simulink model "InductionMachine"  (R2021b)
settings: Solver=FixedStepAuto  StartTime=0.0  StopTime=5  FixedStep=1e-5  RelTol=1e-3
values from neighbouring files (symbols this model uses):
  B = 0.001    [InductionMachine_cal.m]    (also in InductionMachine_dq_cal.m)
  J = 0.2    [InductionMachine_cal.m]    (also in InductionMachine_dq_cal.m)
  L0 = 134.2e-3    (= 0.1342)    [InductionMachine_cal.m]    (also in InductionMachine_dq_cal.m)
  L1 = 135.6e-3    (= 0.1356)    [InductionMachine_cal.m]    (also in InductionMachine_dq_cal.m)
  L2 = 135.6e-3    (= 0.1356)    [InductionMachine_cal.m]    (also in InductionMachine_dq_cal.m)
  omegaSuply = 120 * pi    (= 376.991118431)    [InductionMachine_cal.m]
  P = 4    [InductionMachine_cal.m]    (also in InductionMachine_dq_cal.m)
  R1 = .75    (= 0.75)    [InductionMachine_cal.m]    (also in InductionMachine_dq_cal.m)
  R2 = .46    (= 0.46)    [InductionMachine_cal.m]    (also in InductionMachine_dq_cal.m)
  Tl = 0    [InductionMachine_cal.m]    (also in InductionMachine_dq_cal.m)
  Vsupply = 163    [InductionMachine_cal.m]
Description:
  | Exercise 03 - Lecture 09
settings Model: Creator=Dinh-Tuyen Le  LastModifiedBy=Dinh-Tuyen Le

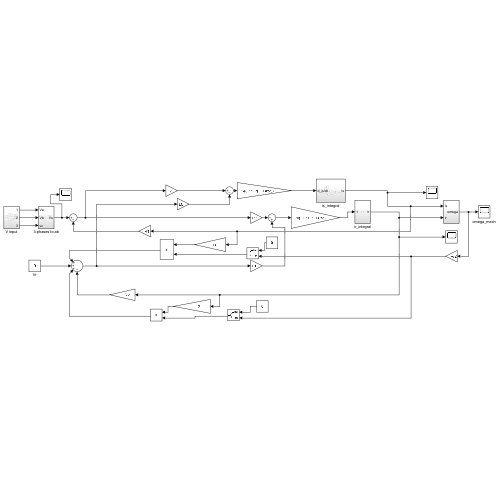
[thumbnail: Simulink's stored preview of the top-level diagram]
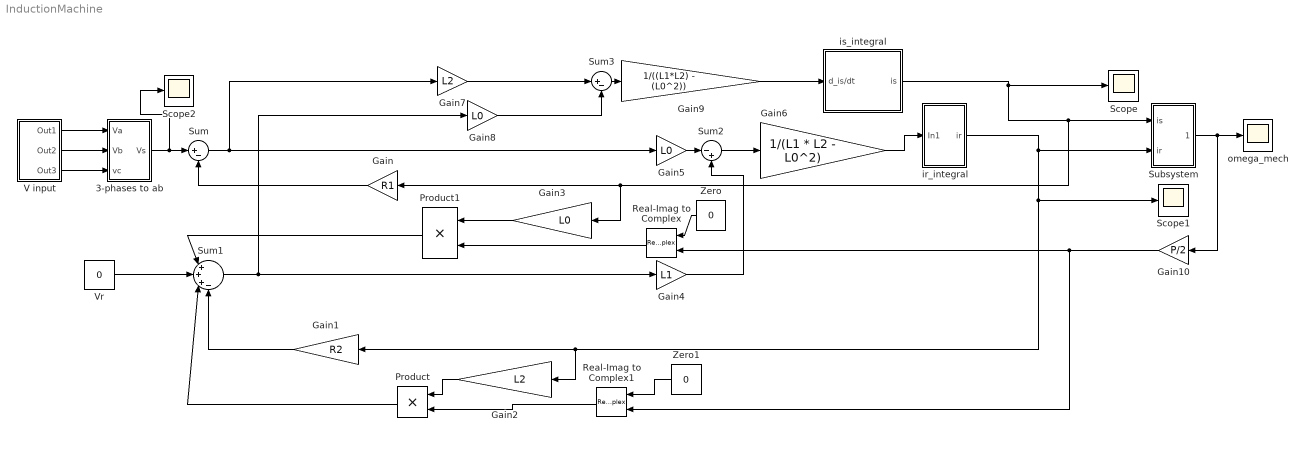
== system InductionMachine ==
  3-phases to ab : Subsystem
  Gain : Gain  Gain=R1
  Gain1 : Gain  Gain=R2
  Gain10 : Gain  Gain=P/2
  Gain2 : Gain  Gain=L2
  Gain3 : Gain  Gain=L0
  Gain4 : Gain  Gain=L1
  Gain5 : Gain  Gain=L0
  Gain6 : Gain  Gain=1/(L1 * L2 - L0^2)
  Gain7 : Gain  Gain=L2
  Gain8 : Gain  Gain=L0
  Gain9 : Gain  Gain=1/((L1*L2) - (L0^2))
  Product : Product
  Product1 : Product
  Real-Imag to Complex : RealImagToComplex
  Real-Imag to Complex1 : RealImagToComplex
  Scope : Scope
  Scope1 : Scope
  Scope2 : Scope
  Subsystem : Subsystem
  Sum : Sum  Inputs=|+-
  Sum1 : Sum  Inputs=|+++-
  Sum2 : Sum  Inputs=|-+
  Sum3 : Sum  Inputs=|+-
  V input : Subsystem
  Vr : Constant  Value=0  OutDataTypeStr=Inherit: Inherit via back propagation
  Zero : Constant  Value=0  OutDataTypeStr=Inherit: Inherit via back propagation
  Zero1 : Constant  Value=0  OutDataTypeStr=Inherit: Inherit via back propagation
  ir_integral : Subsystem
  is_integral : Subsystem
  omega_mech : Scope
  wires:
  Gain/1 -> Sum/2
  Gain1/1 -> Sum1/4
  Vr/1 -> Sum1/2
  Sum1/1 -> Gain8/1, Gain4/1
  Sum/1 -> Gain5/1, Gain7/1
  Gain5/1 -> Sum2/1
  Gain4/1 -> Sum2/2
  Sum2/1 -> Gain6/1
  Gain7/1 -> Sum3/1
  Gain8/1 -> Sum3/2
  Sum3/1 -> Gain9/1
  3-phases to ab/1(Vs) -> Sum/1, Scope2/1
  Subsystem/1(omega) -> omega_mech/1, Gain10/1
  ir_integral/1(ir) -> Gain2/1, Gain1/1, Scope1/1, Subsystem/2(ir)
  Gain6/1 -> ir_integral/1(In1)
  is_integral/1(is) -> Gain/1, Gain3/1, Subsystem/1(is), Scope/1
  Gain9/1 -> is_integral/1(d_is/dt)
  Gain2/1 -> Product/1
  Product/1 -> Sum1/3
  Gain3/1 -> Product1/1
  Product1/1 -> Sum1/1
  Real-Imag to Complex/1 -> Product1/2
  Zero/1 -> Real-Imag to Complex/1
  Zero1/1 -> Real-Imag to Complex1/1
  Real-Imag to Complex1/1 -> Product/2
  V input/1(Out1) -> 3-phases to ab/1(Va)
  V input/2(Out2) -> 3-phases to ab/2(Vb)
  V input/3(Out3) -> 3-phases to ab/3(vc)
  Gain10/1 -> Real-Imag to Complex1/2, Real-Imag to Complex/2

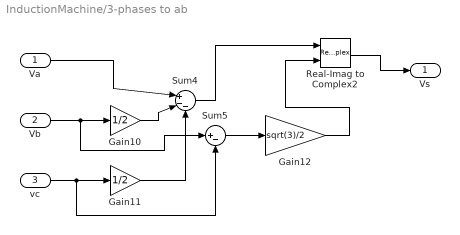
== system InductionMachine/3-phases to ab ==
  Va : Inport
  Vb : Inport  Port=2
  vc : Inport  Port=3
  Gain10 : Gain  Gain=1/2
  Gain11 : Gain  Gain=1/2
  Gain12 : Gain  Gain=sqrt(3)/2
  Real-Imag to Complex2 : RealImagToComplex
  Sum4 : Sum  Inputs=|+--
  Sum5 : Sum  Inputs=|+-
  Vs : Outport
  wires:
  Gain12/1 -> Real-Imag to Complex2/2
  Vb/1 -> Sum5/1, Gain10/1
  Va/1 -> Sum4/1
  Sum4/1 -> Real-Imag to Complex2/1
  Sum5/1 -> Gain12/1
  vc/1 -> Sum5/2, Gain11/1
  Gain11/1 -> Sum4/3
  Gain10/1 -> Sum4/2
  Real-Imag to Complex2/1 -> Vs/1

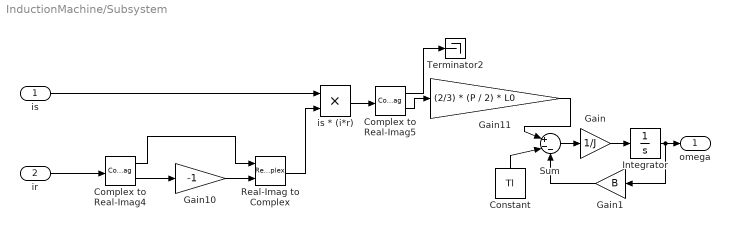
== system InductionMachine/Subsystem ==
  is : Inport
  ir : Inport  Port=2
  Complex to Real-Imag4 : ComplexToRealImag
  Complex to Real-Imag5 : ComplexToRealImag
  Constant : Constant  Value=Tl
  Gain : Gain  Gain=1/J
  Gain1 : Gain  Gain=B
  Gain10 : Gain  Gain=-1
  Gain11 : Gain  Gain=(2/3) * (P / 2) * L0
  Integrator : Integrator
  Real-Imag to Complex : RealImagToComplex
  Sum : Sum  Inputs=|+--
  Terminator2 : Terminator
  is * (i*r) : Product
  omega : Outport
  wires:
  Complex to Real-Imag5/1 -> Terminator2/1
  Complex to Real-Imag5/2 -> Gain11/1
  is * (i*r)/1 -> Complex to Real-Imag5/1
  Real-Imag to Complex/1 -> is * (i*r)/2
  is/1 -> is * (i*r)/1
  Complex to Real-Imag4/1 -> Real-Imag to Complex/1
  Gain10/1 -> Real-Imag to Complex/2
  Complex to Real-Imag4/2 -> Gain10/1
  ir/1 -> Complex to Real-Imag4/1
  Gain11/1 -> Sum/1
  Constant/1 -> Sum/2
  Gain/1 -> Integrator/1
  Integrator/1 -> Gain1/1, omega/1
  Sum/1 -> Gain/1
  Gain1/1 -> Sum/3

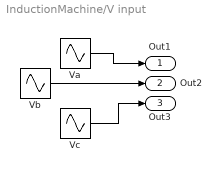
== system InductionMachine/V input ==
  Va : Sin  Amplitude=Vsupply  Frequency=omegaSuply  SampleTime=0
  Vb : Sin  Amplitude=Vsupply  Frequency=omegaSuply  Phase=- 2 * pi / 3  SampleTime=0
  Vc : Sin  Amplitude=Vsupply  Frequency=omegaSuply  Phase=- 4 * pi / 3  SampleTime=0
  Out1 : Outport
  Out2 : Outport  Port=2
  Out3 : Outport  Port=3
  wires:
  Va/1 -> Out1/1
  Vc/1 -> Out3/1
  Vb/1 -> Out2/1

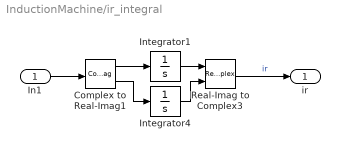
== system InductionMachine/ir_integral ==
  In1 : Inport
  Complex to Real-Imag1 : ComplexToRealImag
  Integrator1 : Integrator
  Integrator4 : Integrator
  Real-Imag to Complex3 : RealImagToComplex
  ir : Outport
  wires:
  Complex to Real-Imag1/1 -> Integrator1/1
  Integrator1/1 -> Real-Imag to Complex3/1
  Complex to Real-Imag1/2 -> Integrator4/1
  Integrator4/1 -> Real-Imag to Complex3/2
  Real-Imag to Complex3/1 -> ir/1  "ir"
  In1/1 -> Complex to Real-Imag1/1

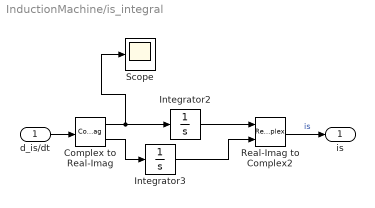
== system InductionMachine/is_integral ==
  d_is/dt : Inport
  Complex to Real-Imag : ComplexToRealImag
  Integrator2 : Integrator
  Integrator3 : Integrator
  Real-Imag to Complex2 : RealImagToComplex
  Scope : Scope
  is : Outport
  wires:
  d_is/dt/1 -> Complex to Real-Imag/1
  Integrator3/1 -> Real-Imag to Complex2/2
  Complex to Real-Imag/2 -> Integrator3/1
  Integrator2/1 -> Real-Imag to Complex2/1
  Real-Imag to Complex2/1 -> is/1  "is"
  Complex to Real-Imag/1 -> Scope/1, Integrator2/1
